simulink model "position_control_motor_wu_bt_sm"  (R2023b)
settings: Solver=FixedStepAuto  StartTime=0.0  StopTime=inf  RelTol=1e-3  EnableMultiTasking=on
undefined symbols (not defined in the file): DiscIntNeverNeededParam, K, Ts
libraries: mbedblockslib x5, cstblocks x1, stm_qeplib x1
settings Model: ExtModeTrigDuration=10  Creator=miche  LastModifiedBy=miche
settings OptimizationCC: EnhancedBackFolding=on  PassReuseOutputArgsAs=Individual arguments  ZeroExternalMemoryAtStartup=off  ZeroInternalMemoryAtStartup=off  MaxStackSize=64  OptimizeBlockOrder=speed  DifferentSizesBufferReuse=on  OptimizationCustomize=off  EfficientTunableParamExpr=on
settings DebuggingCC: ParameterTunabilityLossMsg=error
settings HardwareCC: ProdBitPerPointer=32  ProdBitPerSizeT=32  ProdBitPerPtrDiffT=32  ProdLargestAtomicInteger=Long  ProdLargestAtomicFloat=Double  ProdWordSize=32  ProdLongLongMode=on  ProdHWDeviceType=ARM Compatible->ARM Cortex
settings SFSimCC: MATLABDynamicMemAlloc=off
settings RTWCC: Description=Embedded Coder  SystemTargetFile=ert.tlc  HardwareBoard=STM32 Nucleo F401RE  TemplateMakefile=ert_default_tmf  Toolchain=GNU Tools for ARM Embedded Processors
settings CodeAppCC: ForceParamTrailComments=on  IgnoreCustomStorageClasses=off  OperatorAnnotations=on  SimulinkDataObjDesc=on  SFDataObjDesc=on  InsertBlockDesc=on
settings ERTTargetCC: ExtModeTransport=3  ExtModeStaticAlloc=on  ExtModeStaticAllocSize=2000  ExtModeMexFile=ext_xcp  ExtModeIntrfLevel=Level2 - Open

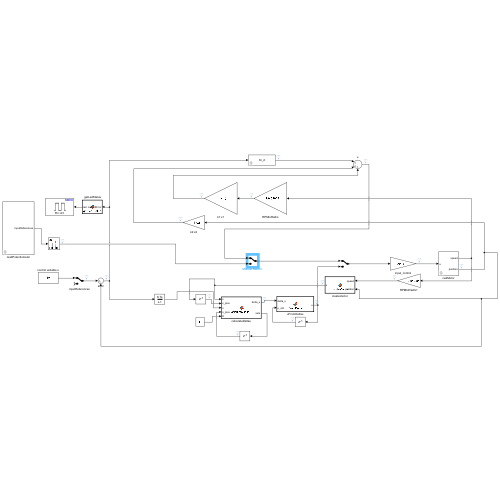
[thumbnail: Simulink's stored preview of the top-level diagram]
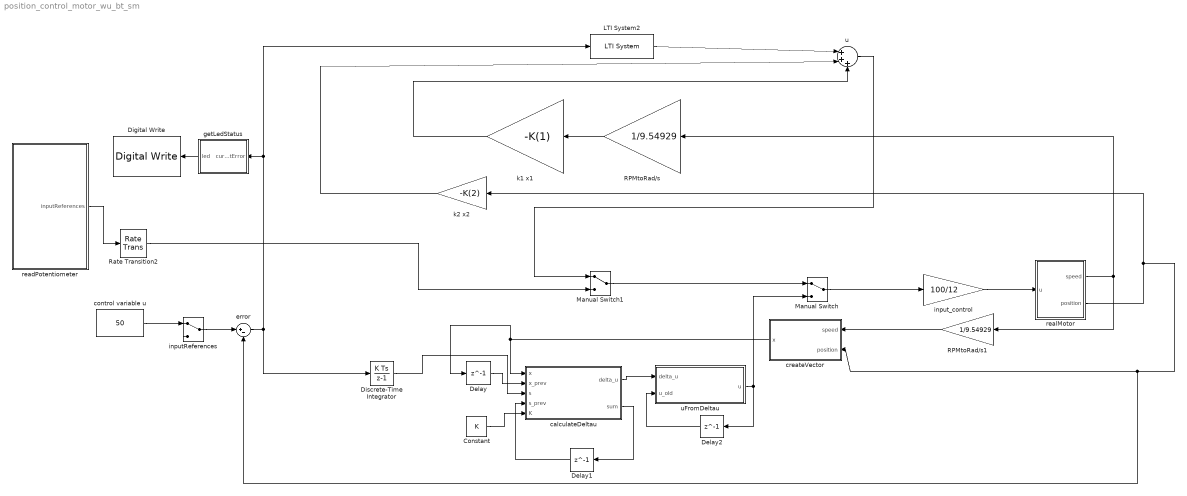
== system position_control_motor_wu_bt_sm ==
  " getLedStatus" : MATLAB Function  TreatAsAtomicUnit=on
  Constant : Constant  Value=K
  Delay : Delay  DelayLength=1  InitialCondition=0  SampleTime=Ts
  Delay1 : Delay  DelayLength=1  InitialCondition=0  SampleTime=Ts
  Delay2 : Delay  DelayLength=1  InitialCondition=0  SampleTime=Ts
  Digital Write : mbedblockslib/Digital Write  Pin=A3  Direction=output
      settings: LibrarySourceBlock=stmnucleorootlib/Common/Digital Write
  Discrete-Time Integrator : DiscreteIntegrator  SampleTime=-1  ICPrevOutput=DiscIntNeverNeededParam  ICPrevScaledInput=DiscIntNeverNeededParam
  LTI System2 : cstblocks/LTI System  sys=Ki_d  IC=[]  PadeOrder=0
  Manual Switch : ManualSwitch
  Manual Switch1 : ManualSwitch
  RPMtoRad/s : Gain  Gain=1/9.54929
  RPMtoRad/s1 : Gain  Gain=1/9.54929
  Rate Transition2 : RateTransition
  calculateDeltau : MATLAB Function  TreatAsAtomicUnit=on
  control variable u : Constant  Value=50
  createVector : MATLAB Function  TreatAsAtomicUnit=on
  error : Sum  Inputs=|+-
  inputReferences : ManualSwitch
  input_control : Gain  Gain=100/12
  k1 x1 : Gain  Gain=-K(1)
  k2 x2 : Gain  Gain=-K(2)
  readPotentiometer : Subsystem  mask{alpha=0.9}
  realMotor : Subsystem  mask{Ts=0.005}
      mask prompts: Ts "sample_time"
  u : Sum  Inputs=|+++
  uFromDeltau : MATLAB Function  TreatAsAtomicUnit=on
  wires:
  control variable u/1 -> inputReferences/1
  inputReferences/1 -> error/1
  " getLedStatus"/1(led) -> Digital Write/1
  realMotor/1(speed) -> RPMtoRad/s/1, RPMtoRad/s1/1
  input_control/1 -> realMotor/1(u)
  readPotentiometer/1(inputReferences) -> Rate Transition2/1
  realMotor/2(position) -> error/2, createVector/2(position), k2 x2/1
  Delay/1 -> calculateDeltau/2(x_prev)
  createVector/1(x) -> calculateDeltau/1(x), Delay/1
  Constant/1 -> calculateDeltau/5(K)
  calculateDeltau/2(sum) -> Delay1/1
  Delay1/1 -> calculateDeltau/4(s_prev)
  calculateDeltau/1(delta_u) -> uFromDeltau/1(delta_u)
  uFromDeltau/1(u) -> Delay2/1, Manual Switch/2
  Delay2/1 -> uFromDeltau/2(u_old)
  RPMtoRad/s1/1 -> createVector/1(speed)
  Discrete-Time Integrator/1 -> calculateDeltau/3(s)
  Rate Transition2/1 -> Manual Switch1/2
  error/1 -> LTI System2/1, " getLedStatus"/1(currentError), Discrete-Time Integrator/1
  LTI System2/1 -> u/1
  RPMtoRad/s/1 -> k1 x1/1
  k2 x2/1 -> u/2
  k1 x1/1 -> u/3
  Manual Switch/1 -> input_control/1
  Manual Switch1/1 -> Manual Switch/1
  u/1 -> Manual Switch1/1

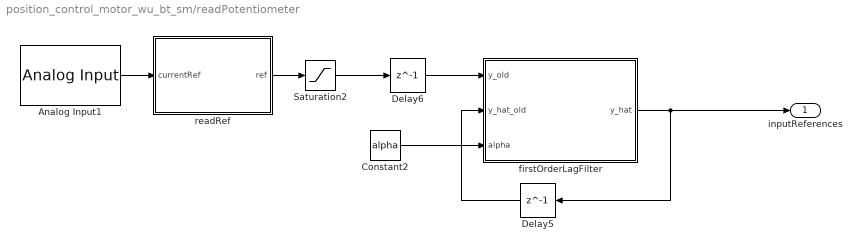
== system position_control_motor_wu_bt_sm/readPotentiometer ==
  Analog Input1 : mbedblockslib/Analog Input  Pin=A4  ReadResultsOnly=off  ConversionTriggerSource=Software  ExternalTriggerType=uint32( 0 )  OutputDataType=double  EnableConversionCompleteNotify=off  EnableOuputStatus=off  SampleTime=0.005/20
      settings: LibrarySourceBlock=stmnucleorootlib/Common/Analog Input
  Constant2 : Constant  Value=alpha
  Delay5 : Delay  DelayLength=1  InitialCondition=0
  Delay6 : Delay  DelayLength=1  InitialCondition=0
  Saturation2 : Saturate  UpperLimit=100  LowerLimit=0
  firstOrderLagFilter : MATLAB Function  TreatAsAtomicUnit=on
  readRef : MATLAB Function  TreatAsAtomicUnit=on
  inputReferences : Outport
  wires:
  Saturation2/1 -> Delay6/1
  Delay6/1 -> firstOrderLagFilter/1(y_old)
  readRef/1(ref) -> Saturation2/1
  Constant2/1 -> firstOrderLagFilter/3(alpha)
  Delay5/1 -> firstOrderLagFilter/2(y_hat_old)
  firstOrderLagFilter/1(y_hat) -> inputReferences/1, Delay5/1
  Analog Input1/1 -> readRef/1(currentRef)

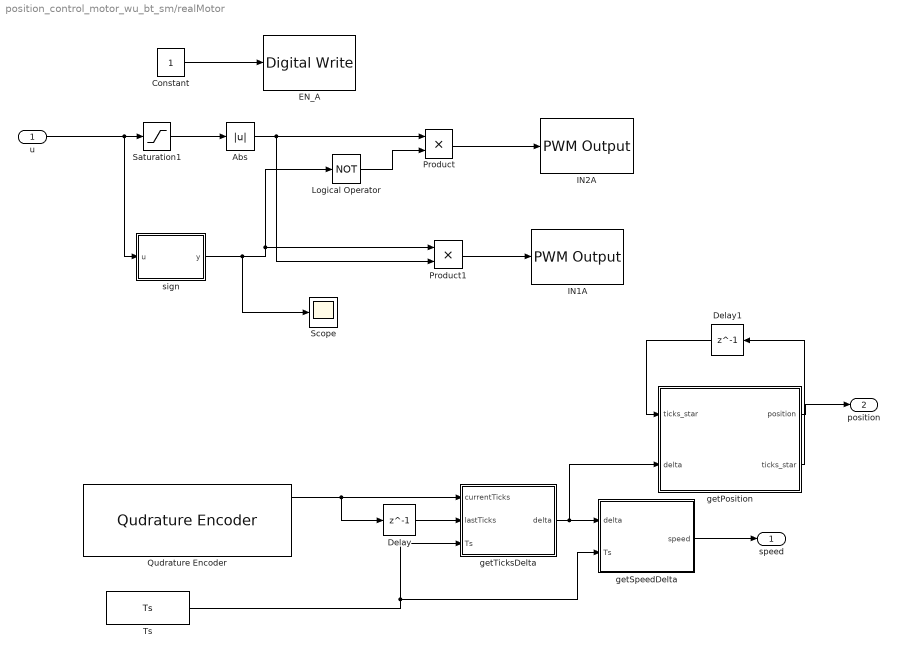
== system position_control_motor_wu_bt_sm/realMotor ==
  u : Inport
  Abs : Abs  SaturateOnIntegerOverflow=off
  Constant : Constant
  Delay : Delay  DelayLength=1  InitialCondition=0
  Delay1 : Delay  DelayLength=1  InitialCondition=0
  EN_A : mbedblockslib/Digital Write  Pin=2  Direction=output
      settings: LibrarySourceBlock=stmnucleorootlib/Common/Digital Write
  IN1A : mbedblockslib/PWM Output  Pin=5  EnableInputFrequency=off  InitialFrequency=2000  InitialDutyCycle=50  NotificationType=None
      settings: LibrarySourceBlock=stmnucleorootlib/Common/PWM Output
  IN2A : mbedblockslib/PWM Output  Pin=4  EnableInputFrequency=off  InitialFrequency=2000  InitialDutyCycle=50  NotificationType=None
      settings: LibrarySourceBlock=stmnucleorootlib/Common/PWM Output
  Logical Operator : Logic  Operator=NOT  AllPortsSameDT=off  OutDataTypeStr=boolean
  Product : Product
  Product1 : Product
  Qudrature Encoder : stm_qeplib/Qudrature Encoder  SampleTime=0.005
  Saturation1 : Saturate  UpperLimit=100  LowerLimit=-100
  Scope : Scope
  Ts : Constant  Value=Ts
  getPosition : MATLAB Function  TreatAsAtomicUnit=on
  getSpeedDelta : MATLAB Function  TreatAsAtomicUnit=on
  getTicksDelta : MATLAB Function  TreatAsAtomicUnit=on
  sign : MATLAB Function  TreatAsAtomicUnit=on
  speed : Outport
  position : Outport  Port=2
  wires:
  sign/1(y) -> Scope/1, Product1/1, Logical Operator/1
  Ts/1 -> getSpeedDelta/2(Ts), getTicksDelta/3(Ts)
  Qudrature Encoder/1 -> Delay/1, getTicksDelta/1(currentTicks)
  Delay1/1 -> getPosition/1("ticks_star ")
  Constant/1 -> EN_A/1
  getPosition/2(ticks_star) -> Delay1/1
  getTicksDelta/1(delta) -> getPosition/2(delta), getSpeedDelta/1(delta)
  Abs/1 -> Product1/2, Product/1
  Product/1 -> IN2A/1
  Logical Operator/1 -> Product/2
  Product1/1 -> IN1A/1
  Delay/1 -> getTicksDelta/2(lastTicks)
  Saturation1/1 -> Abs/1
  getPosition/1(position) -> position/1
  u/1 -> sign/1(u), Saturation1/1
  getSpeedDelta/1(speed) -> speed/1

== matlab function position_control_motor_wu_bt_sm/realMotor/getTicksDelta ==
  data: currentTicks input; delta output; lastTicks input; Ts input
function delta = getTicksDelta(currentTicks,lastTicks, Ts)

currentTicks=double(currentTicks);
lastTicks=double(lastTicks);

if abs(currentTicks -lastTicks) <= ceil(12600*Ts)
    delta= currentTicks - lastTicks;
else
    if lastTicks > currentTicks
        delta= currentTicks + 2^16 -1 - lastTicks;
    else
        delta= currentTicks - 2^16 +1 - lastTicks;
    end
end

end

== matlab function position_control_motor_wu_bt_sm/realMotor/sign ==
  data: u input; y output
function y = sign(u)
if u >0
    y=1;
else
   y=0;
end

== matlab function position_control_motor_wu_bt_sm/realMotor/getSpeedDelta ==
  data: delta input; speed output; Ts input
function speed=getSpeedDelta(delta,Ts)
speed=delta * 60/ (8400*Ts);
end

== matlab function position_control_motor_wu_bt_sm/readPotentiometer/readRef ==
  data: currentRef input; ref output
function ref= readRef(currentRef) 
    
    ref = currentRef * 100
end

== matlab function position_control_motor_wu_bt_sm/realMotor/getPosition ==
  data: ticks_star input; delta input; position output; ticks_star output
function [position,ticks_star] = getPosition(ticks_star, delta)
    ticks_star=double(ticks_star + delta);
    completeTheta=2*pi*ticks_star/(8400);
    position=completeTheta
    %position=sign(completeTheta)*mod(abs(completeTheta), 2*pi)
end

== matlab function position_control_motor_wu_bt_sm/ getLedStatus ==
  data: currentError input; led output
function led = getLedStatus(currentError) 

    if abs(currentError) < 0.1
        led = true;
    else
        led = false;
    end


end

== matlab function position_control_motor_wu_bt_sm/readPotentiometer/firstOrderLagFilter ==
  data: y_old input; y_hat output; y_hat_old input; alpha input
function y_hat = firstOrderLagFilter(y_old, y_hat_old, alpha)
    y_hat= (alpha *y_hat_old) + ((1-alpha)* y_old)
end

== matlab function position_control_motor_wu_bt_sm/calculateDeltau ==
  data: x input; x_prev input; s input; s_prev input; K input; delta_u output; sum output
function [delta_u, sum]= calculateDeltau(x, x_prev, s, s_prev, K)
sum=s;

K1=K(1);
K2=K(2);
K_i=K(3);

delta_x = (x-x_prev);
delta_s = (s-s_prev);

a = -[K1 K2]* delta_x;

b = -K_i*delta_s

delta_u = a+b;

== matlab function position_control_motor_wu_bt_sm/uFromDeltau ==
  data: delta_u input; u_old input; u output
function u = uFromDeltau(delta_u, u_old)
    u = u_old+delta_u;
    if u < -12
        u=-12
    end
    if u > 12
        u=12
    end

== matlab function position_control_motor_wu_bt_sm/createVector ==
  data: speed input; x output; position input
function x = createVector(speed,position)

x = [speed; position];
